simulink model "Drone_fuck_around"  (R2022a)
settings: Solver=VariableStepAuto  StartTime=0.0  StopTime=1  RelTol=1e-7  AbsTol=1e-8
model workspace: external: MATLAB File C:\Users\ivanb\OneDrive\Documents\Team 2261 Files\Mechanical Simulation\DroneMk1_DataFile1.m (data not in the file)
values from neighbouring files (symbols this model uses):
  smiData = saveVarsMat.smiData    [DroneMk1_DataFile1.m]    (also in DroneMk1_DataFile1.mat = )
undefined symbols (not defined in the file or in its folder): X, Y, Z
libraries: sm_lib x42, nesl_utility x30
(part 1 of 2)
settings Model: Creator=ivanb  LastModifiedBy=ivanb
settings SolverCC: InitialStep=1e-8  ZeroCrossAlgorithm=Adaptive

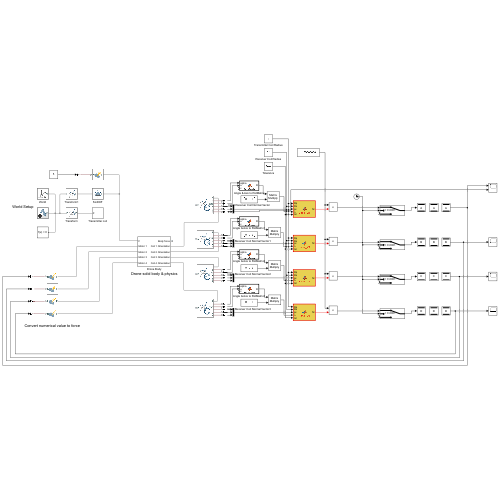
[thumbnail: Simulink's stored preview of the top-level diagram]
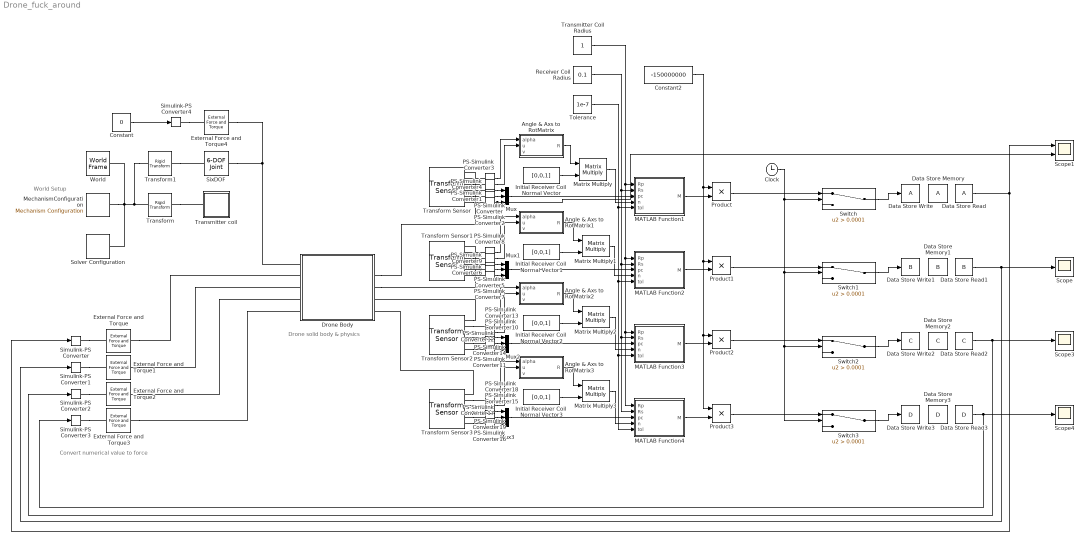
== system Drone_fuck_around ==
  note: Drone solid body & physics
  note: World Setup
  note: Convert numerical value to force
  Angle & Axs to RotMatrix : MATLAB Function  TreatAsAtomicUnit=on
  Angle & Axs to RotMatrix1 : MATLAB Function  TreatAsAtomicUnit=on
  Angle & Axs to RotMatrix2 : MATLAB Function  TreatAsAtomicUnit=on
  Angle & Axs to RotMatrix3 : MATLAB Function  TreatAsAtomicUnit=on
  Clock : Clock
  Constant : Constant  Value=0
  Constant2 : Constant  Value=-150000000
  Data Store Memory : DataStoreMemory  WriteAfterWriteMsg=warning  ShowAdditionalParam=off
  Data Store Memory1 : DataStoreMemory  DataStoreName=B  WriteAfterWriteMsg=warning  ShowAdditionalParam=off
  Data Store Memory2 : DataStoreMemory  DataStoreName=C  WriteAfterWriteMsg=warning  ShowAdditionalParam=off
  Data Store Memory3 : DataStoreMemory  DataStoreName=D  WriteAfterWriteMsg=warning  ShowAdditionalParam=off
  Data Store Read : DataStoreRead  IndexOptions=Index vector (dialog)  Indices=1  OutputSizes=1
  Data Store Read1 : DataStoreRead  DataStoreName=B  IndexOptions=Index vector (dialog)  Indices=1  OutputSizes=1
  Data Store Read2 : DataStoreRead  DataStoreName=C  IndexOptions=Index vector (dialog)  Indices=1  OutputSizes=1
  Data Store Read3 : DataStoreRead  DataStoreName=D  IndexOptions=Index vector (dialog)  Indices=1  OutputSizes=1
  Data Store Write : DataStoreWrite  IndexOptions=Index vector (dialog)  Indices=1  OutputSizes=1
  Data Store Write1 : DataStoreWrite  DataStoreName=B  IndexOptions=Index vector (dialog)  Indices=1  OutputSizes=1
  Data Store Write2 : DataStoreWrite  DataStoreName=C  IndexOptions=Index vector (dialog)  Indices=1  OutputSizes=1
  Data Store Write3 : DataStoreWrite  DataStoreName=D  IndexOptions=Index vector (dialog)  Indices=1  OutputSizes=1
  Drone Body : Subsystem
  External Force and Torque{,1..3} (4 alike) : sm_lib/Forces and Torques/External Force and Torque  ForceResolutionFrame=AttachedFrame  EnableForceX=off  EnableForceY=off  EnableForceZ=on  EnableForce=off  TorqueResolutionFrame=AttachedFrame  EnableTorqueX=off  EnableTorqueY=off  EnableTorqueZ=off  EnableTorque=off
  External Force and Torque4 : sm_lib/Forces and Torques/External Force and Torque  ForceResolutionFrame=AttachedFrame  EnableForceX=off  EnableForceY=off  EnableForceZ=off  EnableForce=off  TorqueResolutionFrame=AttachedFrame  EnableTorqueX=off  EnableTorqueY=on  EnableTorqueZ=off  EnableTorque=off
  Initial Receiver Coil Normal Vector{,1..3} (4 alike) : Constant  Value=[0,0,1]
  MATLAB Function1 : MATLAB Function  TreatAsAtomicUnit=on
  MATLAB Function2 : MATLAB Function  TreatAsAtomicUnit=on
  MATLAB Function3 : MATLAB Function  TreatAsAtomicUnit=on
  MATLAB Function4 : MATLAB Function  TreatAsAtomicUnit=on
  Matrix Multiply{,1..3} (4 alike) : Product  Multiplication=Matrix(*)
  MechanismConfiguration : sm_lib/Utilities/Mechanism Configuration  UniformGravity=Constant  GravityVector=[0 0 -9.80665]  GravityUnits=m/s^2  LinearizationDelta=0.001  JointModeTransitionNonlinearIterations=2
  Mux{,1..3} (4 alike) : Mux  Inputs=3
  PS-Simulink Converter{,1..19} (20 alike) : nesl_utility/PS-Simulink Converter  PhysicalDomain=network_engine_domain  SubClassName=ps_output  LeftPortType=input  RightPortType=output  PseudoPeriodic=off  Frequencies=[]  VectorFormat=inherit  Unit=inherit  AffineConversion=off
      settings: SourceProductBaseCode=SS,PW,VE
  Product{,1..3} (4 alike) : Product
  Receiver Coil Radius : Constant  Value=0.1
  Scope : Scope
  Scope1 : Scope  NumInputPorts=2
  Scope3 : Scope
  Scope4 : Scope
  Simulink-PS Converter{,1..4} (5 alike) : nesl_utility/Simulink-PS Converter  PhysicalDomain=network_engine_domain  SubClassName=ps_input  LeftPortType=input  RightPortType=output  PseudoPeriodic=off  Frequencies=[]  NoiseDistribution=none  NoiseParameters=[]  Unit=1  AffineConversion=off  FilteringAndDerivatives=provide  SimscapeFilterOrder=1  InputFilterTimeConstant=0.001  UdotUserProvided=0
      settings: SourceProductBaseCode=SS,PW,VE
  SixDOF : sm_lib/Joints/6-DOF Joint  JointMode=Normal  SenseConstraintForce=off  SenseConstraintForceX=off  SenseConstraintForceY=off  SenseConstraintForceZ=off  SenseConstraintTorque=off  SenseConstraintTorqueX=off  SenseConstraintTorqueY=off  SenseConstraintTorqueZ=off  SenseTotalForce=off  SenseTotalForceX=off  SenseTotalForceY=off  SenseTotalForceZ=off  SenseTotalTorque=off  SenseTotalTorqueX=off  SenseTotalTorqueY=off  SenseTotalTorqueZ=off  CompositeWrenchDir=FollowerOnBase  CompositeWrenchFrame=BaseFrame  PxEquilibriumPosition=0  PxEquilibriumPositionUnits=m  PxSpringStiffness=0  PxSpringStiffnessUnits=N/m  PxDampingCoefficient=0  PxDampingCoefficientUnits=N/(m/s)  PxTorqueActuationMode=NoTorque  PxMotionActuationMode=ComputedMotion  PxSensePosition=off  PxSenseVelocity=off  PxSenseAcceleration=off  PxSenseTorqueForce=off  PxSenseLowerLimitTorqueForce=off  PxSenseUpperLimitTorqueForce=off  PxLowerLimitSpecify=off  PxLowerLimitBound=-1  PxLowerLimitBoundUnits=m  PxLowerLimitStiffness=1e6  PxLowerLimitStiffnessUnits=N/m  PxLowerLimitDamping=1e3  PxLowerLimitDampingUnits=N/(m/s)  PxLowerLimitTransitionRegionWidth=1e-4  PxLowerLimitTransitionRegionWidthUnits=m  PxUpperLimitSpecify=off  PxUpperLimitBound=1  PxUpperLimitBoundUnits=m  PxUpperLimitStiffness=1e6  PxUpperLimitStiffnessUnits=N/m  PxUpperLimitDamping=1e3  PxUpperLimitDampingUnits=N/(m/s)  PxUpperLimitTransitionRegionWidth=1e-4  PxUpperLimitTransitionRegionWidthUnits=m  PxPositionTargetSpecify=off  PxPositionTargetPriority=High  PxPositionTargetValue=0  PxPositionTargetValueUnits=m  PxVelocityTargetSpecify=off  PxVelocityTargetPriority=High  PxVelocityTargetValue=0.001  PxVelocityTargetValueUnits=m/s  PyEquilibriumPosition=0  PyEquilibriumPositionUnits=m  PySpringStiffness=0  PySpringStiffnessUnits=N/m  PyDampingCoefficient=0  PyDampingCoefficientUnits=N/(m/s)  PyTorqueActuationMode=NoTorque  PyMotionActuationMode=ComputedMotion  PySensePosition=off  PySenseVelocity=off  PySenseAcceleration=off  PySenseTorqueForce=off  PySenseLowerLimitTorqueForce=off  PySenseUpperLimitTorqueForce=off  PyLowerLimitSpecify=off  PyLowerLimitBound=-1  PyLowerLimitBoundUnits=m  PyLowerLimitStiffness=1e6  PyLowerLimitStiffnessUnits=N/m  PyLowerLimitDamping=1e3  PyLowerLimitDampingUnits=N/(m/s)  PyLowerLimitTransitionRegionWidth=1e-4  PyLowerLimitTransitionRegionWidthUnits=m  PyUpperLimitSpecify=off  PyUpperLimitBound=1  PyUpperLimitBoundUnits=m  PyUpperLimitStiffness=1e6  PyUpperLimitStiffnessUnits=N/m  PyUpperLimitDamping=1e3  PyUpperLimitDampingUnits=N/(m/s)  PyUpperLimitTransitionRegionWidth=1e-4  PyUpperLimitTransitionRegionWidthUnits=m  PyPositionTargetSpecify=off  PyPositionTargetPriority=High  PyPositionTargetValue=0  PyPositionTargetValueUnits=m  PyVelocityTargetSpecify=off  PyVelocityTargetPriority=High  PyVelocityTargetValue=0  PyVelocityTargetValueUnits=m/s  PzEquilibriumPosition=0  PzEquilibriumPositionUnits=m  PzSpringStiffness=0  PzSpringStiffnessUnits=N/m  PzDampingCoefficient=0  PzDampingCoefficientUnits=N/(m/s)  PzTorqueActuationMode=NoTorque  PzMotionActuationMode=ComputedMotion  PzSensePosition=off  PzSenseVelocity=off  PzSenseAcceleration=off  PzSenseTorqueForce=off  PzSenseLowerLimitTorqueForce=off  PzSenseUpperLimitTorqueForce=off  PzLowerLimitSpecify=off  PzLowerLimitBound=-1  PzLowerLimitBoundUnits=m  PzLowerLimitStiffness=1e6  PzLowerLimitStiffnessUnits=N/m  PzLowerLimitDamping=1e3  PzLowerLimitDampingUnits=N/(m/s)  PzLowerLimitTransitionRegionWidth=1e-4  PzLowerLimitTransitionRegionWidthUnits=m  PzUpperLimitSpecify=off  PzUpperLimitBound=1  PzUpperLimitBoundUnits=m  PzUpperLimitStiffness=1e6  PzUpperLimitStiffnessUnits=N/m  PzUpperLimitDamping=1e3  PzUpperLimitDampingUnits=N/(m/s)  PzUpperLimitTransitionRegionWidth=1e-4  PzUpperLimitTransitionRegionWidthUnits=m  PzPositionTargetSpecify=off  PzPositionTargetPriority=High  PzPositionTargetValue=0  PzPositionTargetValueUnits=m  PzVelocityTargetSpecify=off  PzVelocityTargetPriority=High  PzVelocityTargetValue=0  PzVelocityTargetValueUnits=m/s  SphDefPosRotationMethod=None  SphDefPosRotationAngleUnits=deg  SphDefPosRotationStandardAxis=+Z  SphDefPosRotationAngle=0.0  SphDefPosRotationArbitraryAxis=[0 0 1]  SphDefPosFollAlignAxisA=+X  SphDefPosBaseAlignAxisA=+Y  SphDefPosFollAlignAxisB=+Y  SphDefPosBaseAlignAxisB=+Z  SphDefPosRotationSequenceAxes=FollowerAxes  SphDefPosRotationSequence=XYX  SphDefPosRotationSequenceAngles=[0 0 0]  SphDefPosRotationSequenceAnglesUnits=deg  SphDefPosRotationMatrix=[1 0 0; 0 1 0; 0 0 1]  SphEqPosRotationMethod=None  SphEqPosRotationAngleUnits=deg  SphEqPosRotationStandardAxis=+Z  SphEqPosRotationAngle=0.0  SphEqPosRotationArbitraryAxis=[0 0 1]  SphEqPosFollAlignAxisA=+X  SphEqPosBaseAlignAxisA=+Y  SphEqPosFollAlignAxisB=+Y  SphEqPosBaseAlignAxisB=+Z  SphEqPosRotationSequenceAxes=FollowerAxes  SphEqPosRotationSequence=XYX  SphEqPosRotationSequenceAngles=[0 0 0]  SphEqPosRotationSequenceAnglesUnits=deg  SphEqPosRotationMatrix=[1 0 0; 0 1 0; 0 0 1]  SphSpringStiffness=0  SphSpringStiffnessUnits=N*m/deg  SphDampingCoefficient=0  SphDampingCoefficientUnits=N*m/(deg/s)  SphActuateTorqueX=off  SphActuateTorqueY=off  SphActuateTorqueZ=off  SphActuateTorque=off  SphTorqueActuationMode=NoTorque  SphMotionActuationMode=ComputedMotion  SphActuationFrame=BaseFrame  SphSensePosition=off  SphSenseVelocityX=off  SphSenseVelocityY=off  SphSenseVelocityZ=off  SphSenseVelocity=off  SphSenseAccelerationX=off  SphSenseAccelerationY=off  SphSenseAccelerationZ=off  SphSenseAcceleration=off  SphSenseTorqueX=off  SphSenseTorqueY=off  SphSenseTorqueZ=off  SphSenseTorqueForce=off  SphSenseLowerLimitTorqueMag=off  SphSenseUpperLimitTorqueMag=off  SphSensingFrame=FollowerFrame  SphLowerLimitSpecify=off  SphLowerLimitBound=15  SphLowerLimitBoundUnits=deg  SphLowerLimitStiffness=1e4  SphLowerLimitStiffnessUnits=N*m/deg  SphLowerLimitDamping=10  SphLowerLimitDampingUnits=N*m/(deg/s)  SphLowerLimitTransitionRegionWidth=0.1  SphLowerLimitTransitionRegionWidthUnits=deg  SphUpperLimitSpecify=off  SphUpperLimitBound=45  SphUpperLimitBoundUnits=deg  SphUpperLimitStiffness=1e4  SphUpperLimitStiffnessUnits=N*m/deg  SphUpperLimitDamping=10  SphUpperLimitDampingUnits=N*m/(deg/s)  SphUpperLimitTransitionRegionWidth=0.1  SphUpperLimitTransitionRegionWidthUnits=deg  SphPositionTargetRotationMethod=None  SphPositionTargetRotationAngleUnits=deg  SphPositionTargetRotationStandardAxis=+Z  SphPositionTargetRotationAngle=0.0  SphPositionTargetRotationArbitraryAxis=[0 0 1]  SphPositionTargetFollAlignAxisA=+X  SphPositionTargetBaseAlignAxisA=+Y  SphPositionTargetFollAlignAxisB=+Y  SphPositionTargetBaseAlignAxisB=+Z  SphPositionTargetRotationSequenceAxes=FollowerAxes  SphPositionTargetRotationSequence=XYX  SphPositionTargetRotationSequenceAngles=[0 0 0]  SphPositionTargetRotationSequenceAnglesUnits=deg  SphPositionTargetRotationMatrix=[1 0 0; 0 1 0; 0 0 1]  SphPositionTargetSpecify=off  SphPositionTargetPriority=High  SphVelocityTargetValue=[0 0 0]  SphVelocityTargetValueUnits=deg/s  SphVelocityTargetSpecify=off  SphVelocityTargetPriority=High  SphVelocityTargetInFollowerFrame=on
  Solver Configuration : nesl_utility/Solver Configuration  PhysicalDomain=network_engine_domain  SubClassName=solver  LeftPortType=input  RightPortType=generic  Tones=[]  Harmonics=[]  SimulateNoise=off  Profile=off  UseLocalSampling=off  EnableSwitchedLinearOptims=on  FrequencyDomain=off  UseCCode=off  RelTol=0.001  AbsTol=0.001  MinStep=1e-09  ToWorkspace=off  RevertToSquareIcSolve=off  NumHomotopyIterations=100  PhasorMode=off  PhasorModeNumHarmonics=1  IndexReductionMethod=DerivativeReplacement  DoDC=off  ResidualTolerance=1e-09  UseLocalSolver=off  LocalSolverChoice=NE_BACKWARD_EULER_ADVANCER  LocalSolverSampleTime=0.001  DoFixedCost=off  MaxNonlinIter=3  MaxModeIter=2  ComputeImpulses=off  ImpulseIterations=2  LinearAlgebra=auto  LinearAlgebraNumThread=0  EquationFormulation=NE_TIME_EF  DelaysMemoryBudget=1024  AutomaticFiltering=on  FilteringTimeConstant=0.001  PartitionStorageMethod=AS_NEEDED  PartitionMemoryBudget=1024  PartitionMethod=ROBUST
      settings: SourceProductBaseCode=SS,PW,VE
  Switch{,1..3} (4 alike) : Switch  Criteria=u2 > Threshold  Threshold=0.0001  SaturateOnIntegerOverflow=off  InputSameDT=off
  Tolerance : Constant  Value=1e-7
  Transform : sm_lib/Frames and Transforms/Rigid Transform  TranslationMethod=Cartesian  TranslationStandardOffset=0  TranslationLengthUnit=m  TranslationStandardAxis=+Z  TranslationCartesianOffset=[0, 0, 0]  TranslationROffset=0  TranslationROffsetUnits=m  TranslationZOffset=0  TranslationZOffsetUnits=m  TranslationThetaOffset=0  TranslationThetaOffsetUnits=deg  RotationMethod=StandardAxis  RotationAngleUnits=rad  RotationStandardAxis=-X  RotationAngle=pi/2  RotationArbitraryAxis=smiData.RigidTransform(1).axis  FollAlignAxisA=+X  BaseAlignAxisA=+Y  FollAlignAxisB=+Y  BaseAlignAxisB=+Z  RotationSequenceAxes=FollowerAxes  RotationSequence=XYX  RotationSequenceAngles=[0 0 0]  RotationSequenceAnglesUnits=deg  RotationMatrix=[1 0 0; 0 1 0; 0 0 1]
  Transform Sensor{,1..3} (4 alike) : sm_lib/Frames and Transforms/Transform Sensor  MeasurementFrame=World  SenseAngle=on  SenseAxis=on  SenseAngle1=off  SenseAngle2=off  SenseAngle3=off  SenseQ=off  SenseR=off  SenseOmegaX=off  SenseOmegaY=off  SenseOmegaZ=off  SenseOmega1=off  SenseOmega2=off  SenseOmega3=off  SenseQDot=off  SenseRDot=off  SenseAlphaX=off  SenseAlphaY=off  SenseAlphaZ=off  SenseAlpha1=off  SenseAlpha2=off  SenseAlpha3=off  SenseQDDot=off  SenseRDDot=off  SenseX=on  SenseY=on  SenseZ=on  SenseRad=off  SenseAzim=off  SenseDist=off  SenseInc=off  SenseXDot=off  SenseYDot=off  SenseZDot=off  SenseRadDot=off  SenseAzimDot=off  SenseDistDot=off  SenseIncDot=off  SenseXDDot=off  SenseYDDot=off  SenseZDDot=off  SenseRadDDot=off  SenseAzimDDot=off  SenseDistDDot=off  SenseIncDDot=off
  Transform1 : sm_lib/Frames and Transforms/Rigid Transform  TranslationMethod=Cartesian  TranslationStandardOffset=0  TranslationLengthUnit=m  TranslationStandardAxis=+Z  TranslationCartesianOffset=[0, 0, 0.1]  TranslationROffset=0  TranslationROffsetUnits=m  TranslationZOffset=0  TranslationZOffsetUnits=m  TranslationThetaOffset=0  TranslationThetaOffsetUnits=deg  RotationMethod=StandardAxis  RotationAngleUnits=rad  RotationStandardAxis=+X  RotationAngle=pi/2  RotationArbitraryAxis=smiData.RigidTransform(2).axis  FollAlignAxisA=+X  BaseAlignAxisA=+Y  FollAlignAxisB=+Y  BaseAlignAxisB=+Z  RotationSequenceAxes=FollowerAxes  RotationSequence=XYX  RotationSequenceAngles=[0 0 0]  RotationSequenceAnglesUnits=deg  RotationMatrix=[1 0 0; 0 1 0; 0 0 1]
  Transmitter Coil Radius : Constant
  Transmitter coil : Subsystem
  World : sm_lib/Frames and Transforms/World Frame
  wires:
  Switch/1 -> Data Store Write/1
  Clock/1 -> Switch3/2, Switch2/2, Switch1/2, Switch/2
  Data Store Read/1 -> Simulink-PS Converter/1, Scope1/1
  Mux3/1 -> MATLAB Function4/3(pc)
  Matrix Multiply1/1 -> MATLAB Function2/4(n)
  Angle & Axs to RotMatrix1/1(R) -> Matrix Multiply1/1
  MATLAB Function2/1(M) -> Product1/2
  PS-Simulink Converter12/1 -> Mux2/3
  PS-Simulink Converter10/1 -> Mux2/1
  Initial Receiver Coil Normal Vector3/1 -> Matrix Multiply3/2
  PS-Simulink Converter3/1 -> Angle & Axs to RotMatrix/1(alpha)
  MATLAB Function3/1(M) -> Product2/2
  PS-Simulink Converter18/1 -> Angle & Axs to RotMatrix3/1(alpha)
  Initial Receiver Coil Normal Vector2/1 -> Matrix Multiply2/2
  Receiver Coil Radius/1 -> MATLAB Function1/2(Rs), MATLAB Function2/2(Rs), MATLAB Function4/2(Rs), MATLAB Function3/2(Rs)
  Tolerance/1 -> MATLAB Function1/5(tol), MATLAB Function2/5(tol), MATLAB Function4/5(tol), MATLAB Function3/5(tol)
  Initial Receiver Coil Normal Vector1/1 -> Matrix Multiply1/2
  MATLAB Function4/1(M) -> Product3/2
  PS-Simulink Converter19/1 -> Angle & Axs to RotMatrix3/2(u)
  Transmitter Coil Radius/1 -> MATLAB Function1/1(Rp), MATLAB Function2/1(Rp), MATLAB Function4/1(Rp), MATLAB Function3/1(Rp)
  Angle & Axs to RotMatrix3/1(R) -> Matrix Multiply3/1
  PS-Simulink Converter6/1 -> Mux1/2
  Initial Receiver Coil Normal Vector/1 -> Matrix Multiply/2
  Matrix Multiply3/1 -> MATLAB Function4/4(n)
  PS-Simulink Converter14/1 -> Angle & Axs to RotMatrix2/2(u)
  PS-Simulink Converter9/1 -> Angle & Axs to RotMatrix1/2(u)
  PS-Simulink Converter7/1 -> Mux1/3
  PS-Simulink Converter13/1 -> Angle & Axs to RotMatrix2/1(alpha)
  PS-Simulink Converter17/1 -> Mux3/3
  PS-Simulink Converter2/1 -> Scope1/2, Mux/3
  PS-Simulink Converter16/1 -> Mux3/2
  PS-Simulink Converter15/1 -> Mux3/1
  Mux2/1 -> MATLAB Function3/3(pc)
  MATLAB Function1/1(M) -> Product/2
  PS-Simulink Converter8/1 -> Angle & Axs to RotMatrix1/1(alpha)
  Mux1/1 -> MATLAB Function2/3(pc)
  Angle & Axs to RotMatrix/1(R) -> Matrix Multiply/1
  PS-Simulink Converter11/1 -> Mux2/2
  Constant/1 -> Simulink-PS Converter4/1
  Mux/1 -> MATLAB Function1/3(pc)
  PS-Simulink Converter4/1 -> Angle & Axs to RotMatrix/2(u)
  Angle & Axs to RotMatrix2/1(R) -> Matrix Multiply2/1
  Matrix Multiply/1 -> MATLAB Function1/4(n)
  PS-Simulink Converter/1 -> Mux/1
  Matrix Multiply2/1 -> MATLAB Function3/4(n)
  PS-Simulink Converter5/1 -> Mux1/1
  Switch1/1 -> Data Store Write1/1
  Switch2/1 -> Data Store Write2/1
  Switch3/1 -> Data Store Write3/1
  Data Store Read1/1 -> Scope/1, Simulink-PS Converter1/1
  Data Store Read2/1 -> Scope3/1, Simulink-PS Converter2/1
  Data Store Read3/1 -> Scope4/1, Simulink-PS Converter3/1
  Constant2/1 -> Product3/1, Product2/1, Product1/1, Product/1
  PS-Simulink Converter1/1 -> Mux/2
  Product/1 -> Switch/1
  Product1/1 -> Switch1/1
  Product2/1 -> Switch2/1
  Product3/1 -> Switch3/1
  connections:
  Transform1/LConn1 -- Transform/LConn1 -- MechanismConfiguration/RConn1 -- Solver Configuration/RConn1 -- World/RConn1
  SixDOF/RConn1 -- Drone Body/LConn1 -- External Force and Torque4/RConn1
  Transform Sensor2/RConn2 -- PS-Simulink Converter13/LConn1
  Transform Sensor3/RConn5 -- PS-Simulink Converter16/LConn1
  Transform Sensor3/RConn3 -- PS-Simulink Converter19/LConn1
  External Force and Torque2/RConn1 -- Drone Body/LConn4
  Transform Sensor3/RConn6 -- PS-Simulink Converter17/LConn1
  Transform Sensor2/RConn1 -- Drone Body/RConn4
  Transform Sensor/RConn3 -- PS-Simulink Converter4/LConn1
  Simulink-PS Converter4/RConn1 -- External Force and Torque4/LConn1
  Drone Body/RConn2 -- Transform Sensor/RConn1
  Simulink-PS Converter3/RConn1 -- External Force and Torque3/LConn1
  Transform Sensor1/RConn2 -- PS-Simulink Converter8/LConn1
  Transform Sensor/RConn2 -- PS-Simulink Converter3/LConn1
  Transform Sensor1/RConn5 -- PS-Simulink Converter6/LConn1
  Transform Sensor2/RConn3 -- PS-Simulink Converter14/LConn1
  Simulink-PS Converter/RConn1 -- External Force and Torque/LConn1
  Transform Sensor/RConn5 -- PS-Simulink Converter1/LConn1
  External Force and Torque3/RConn1 -- Drone Body/LConn5
  Transform Sensor1/RConn3 -- PS-Simulink Converter9/LConn1
  Drone Body/RConn3 -- Transform Sensor1/RConn1
  Transform Sensor3/RConn4 -- PS-Simulink Converter15/LConn1
  Transform Sensor3/RConn2 -- PS-Simulink Converter18/LConn1
  Transform Sensor/RConn6 -- PS-Simulink Converter2/LConn1
  Simulink-PS Converter1/RConn1 -- External Force and Torque1/LConn1
  Transform Sensor1/RConn6 -- PS-Simulink Converter7/LConn1
  Transform Sensor3/RConn1 -- Drone Body/RConn5
  External Force and Torque/RConn1 -- Drone Body/LConn2
  Transform Sensor2/RConn4 -- PS-Simulink Converter10/LConn1
  Transform Sensor/RConn4 -- PS-Simulink Converter/LConn1
  Transform/RConn1 -- Transmitter coil/LConn1
  Transform Sensor2/RConn5 -- PS-Simulink Converter11/LConn1
  Simulink-PS Converter2/RConn1 -- External Force and Torque2/LConn1
  Transform Sensor2/RConn6 -- PS-Simulink Converter12/LConn1
  Transform Sensor1/RConn4 -- PS-Simulink Converter5/LConn1
  External Force and Torque1/RConn1 -- Drone Body/LConn3
  Transform1/RConn1 -- SixDOF/LConn1

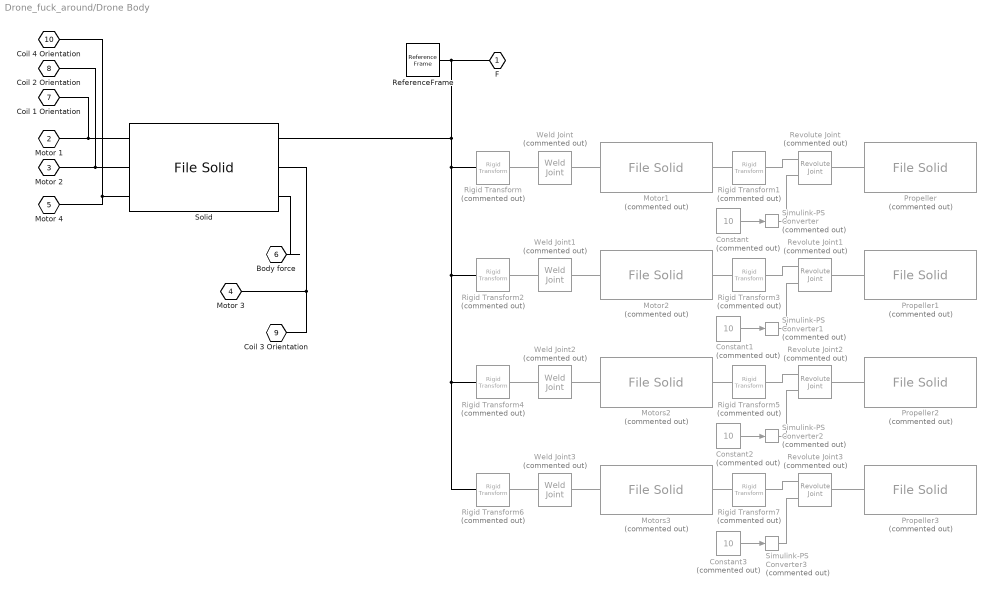
== system Drone_fuck_around/Drone Body ==
  Constant{,1..3} (4 alike) : Constant  Commented=on  Value=10
  Motor1 : sm_lib/Body Elements/File Solid  Commented=on  ExtGeomFileName=C:\Users\ivanb\OneDrive\Documents\Team 2261 Files\Mechanical Simulation\Drone Rendering\Rendered_for_simulink\DC_MOTOR_(Brushless DC Inrunner Motor)_Default_sldprt.STEP  UnitType=FromFile  ExtGeomFileUnits=m  StepReaderType=HEX  ExportConvexHullGeometry=off  InertiaType=CalculateFromGeometry  Mass=1  MassUnits=kg  CenterOfMass=[0 0 0]  CenterOfMassUnits=m  MomentsOfInertia=[1 1 1]  MomentsOfInertiaUnits=kg*m^2  ProductsOfInertia=[0 0 0]  ProductsOfInertiaUnits=kg*m^2  BasedOnType=Density  Density=1000  DensityUnits=kg/m^3  DoExposeReferenceFrame=on  SerializedFrames=<Frames><Frame><Id>Frame1</Id><Value><Name>Position</Name><Origin><Source>ReferenceFrame</Source><FeatureName></FeatureName></Origin><PrimaryAxis><DefinedDirection>+Z</DefinedDirection><Source>ReferenceFrame</Source><SourceDirection>+Z</SourceDirection><FeatureName></FeatureName></PrimaryAxis><SecondaryAxis><DefinedDirection>+X</DefinedDirection><Source>ReferenceFrame</Source><SourceDirection>+X</SourceDirection><FeatureName></FeatureName></SecondaryAxis></Value></Frame></Frames>  GraphicType=FromGeometry  MarkerShape=Sphere  MarkerSize=10  GraphicVisPropType=SimpleVisualProperties  GraphicDiffuseColor=[0.5 0.5 0.5]  GraphicSpecularColor=[0.5 0.5 0.5 1.0]  GraphicAmbientColor=[0.15 0.15 0.15 1.0]  GraphicEmissiveColor=[0.0 0.0 0.0 1.0]  GraphicShininess=75  GraphicOpacity=1.0
  Motor2 : sm_lib/Body Elements/File Solid  Commented=on  ExtGeomFileName=C:\Users\ivanb\OneDrive\Documents\Team 2261 Files\Mechanical Simulation\Drone Rendering\Rendered_for_simulink\DC_MOTOR_(Brushless DC Inrunner Motor)_Default_sldprt.STEP  UnitType=FromFile  ExtGeomFileUnits=m  StepReaderType=HEX  ExportConvexHullGeometry=off  InertiaType=CalculateFromGeometry  Mass=1  MassUnits=kg  CenterOfMass=[0 0 0]  CenterOfMassUnits=m  MomentsOfInertia=[1 1 1]  MomentsOfInertiaUnits=kg*m^2  ProductsOfInertia=[0 0 0]  ProductsOfInertiaUnits=kg*m^2  BasedOnType=Density  Density=1000  DensityUnits=kg/m^3  DoExposeReferenceFrame=on  SerializedFrames=<Frames><Frame><Id>Frame1</Id><Value><Name>Position</Name><Origin><Source>ReferenceFrame</Source><FeatureName></FeatureName></Origin><PrimaryAxis><DefinedDirection>+Z</DefinedDirection><Source>ReferenceFrame</Source><SourceDirection>+Z</SourceDirection><FeatureName></FeatureName></PrimaryAxis><SecondaryAxis><DefinedDirection>+X</DefinedDirection><Source>ReferenceFrame</Source><SourceDirection>+X</SourceDirection><FeatureName></FeatureName></SecondaryAxis></Value></Frame></Frames>  GraphicType=FromGeometry  MarkerShape=Sphere  MarkerSize=10  GraphicVisPropType=SimpleVisualProperties  GraphicDiffuseColor=[0.5 0.5 0.5]  GraphicSpecularColor=[0.5 0.5 0.5 1.0]  GraphicAmbientColor=[0.15 0.15 0.15 1.0]  GraphicEmissiveColor=[0.0 0.0 0.0 1.0]  GraphicShininess=75  GraphicOpacity=1.0
  Motors2 : sm_lib/Body Elements/File Solid  Commented=on  ExtGeomFileName=C:\Users\ivanb\OneDrive\Documents\Team 2261 Files\Mechanical Simulation\Drone Rendering\Rendered_for_simulink\DC_MOTOR_(Brushless DC Inrunner Motor)_Default_sldprt.STEP  UnitType=FromFile  ExtGeomFileUnits=m  StepReaderType=HEX  ExportConvexHullGeometry=off  InertiaType=CalculateFromGeometry  Mass=1  MassUnits=kg  CenterOfMass=[0 0 0]  CenterOfMassUnits=m  MomentsOfInertia=[1 1 1]  MomentsOfInertiaUnits=kg*m^2  ProductsOfInertia=[0 0 0]  ProductsOfInertiaUnits=kg*m^2  BasedOnType=Density  Density=1000  DensityUnits=kg/m^3  DoExposeReferenceFrame=on  SerializedFrames=<Frames><Frame><Id>Frame1</Id><Value><Name>Position</Name><Origin><Source>ReferenceFrame</Source><FeatureName></FeatureName></Origin><PrimaryAxis><DefinedDirection>+Z</DefinedDirection><Source>ReferenceFrame</Source><SourceDirection>+Z</SourceDirection><FeatureName></FeatureName></PrimaryAxis><SecondaryAxis><DefinedDirection>+X</DefinedDirection><Source>ReferenceFrame</Source><SourceDirection>+X</SourceDirection><FeatureName></FeatureName></SecondaryAxis></Value></Frame></Frames>  GraphicType=FromGeometry  MarkerShape=Sphere  MarkerSize=10  GraphicVisPropType=SimpleVisualProperties  GraphicDiffuseColor=[0.5 0.5 0.5]  GraphicSpecularColor=[0.5 0.5 0.5 1.0]  GraphicAmbientColor=[0.15 0.15 0.15 1.0]  GraphicEmissiveColor=[0.0 0.0 0.0 1.0]  GraphicShininess=75  GraphicOpacity=1.0
  Motors3 : sm_lib/Body Elements/File Solid  Commented=on  ExtGeomFileName=C:\Users\ivanb\OneDrive\Documents\Team 2261 Files\Mechanical Simulation\Drone Rendering\Rendered_for_simulink\DC_MOTOR_(Brushless DC Inrunner Motor)_Default_sldprt.STEP  UnitType=FromFile  ExtGeomFileUnits=m  StepReaderType=HEX  ExportConvexHullGeometry=off  InertiaType=CalculateFromGeometry  Mass=1  MassUnits=kg  CenterOfMass=[0 0 0]  CenterOfMassUnits=m  MomentsOfInertia=[1 1 1]  MomentsOfInertiaUnits=kg*m^2  ProductsOfInertia=[0 0 0]  ProductsOfInertiaUnits=kg*m^2  BasedOnType=Density  Density=1000  DensityUnits=kg/m^3  DoExposeReferenceFrame=on  SerializedFrames=<Frames><Frame><Id>Frame1</Id><Value><Name>Position</Name><Origin><Source>ReferenceFrame</Source><FeatureName></FeatureName></Origin><PrimaryAxis><DefinedDirection>+Z</DefinedDirection><Source>ReferenceFrame</Source><SourceDirection>+Z</SourceDirection><FeatureName></FeatureName></PrimaryAxis><SecondaryAxis><DefinedDirection>+X</DefinedDirection><Source>ReferenceFrame</Source><SourceDirection>+X</SourceDirection><FeatureName></FeatureName></SecondaryAxis></Value></Frame></Frames>  GraphicType=FromGeometry  MarkerShape=Sphere  MarkerSize=10  GraphicVisPropType=SimpleVisualProperties  GraphicDiffuseColor=[0.5 0.5 0.5]  GraphicSpecularColor=[0.5 0.5 0.5 1.0]  GraphicAmbientColor=[0.15 0.15 0.15 1.0]  GraphicEmissiveColor=[0.0 0.0 0.0 1.0]  GraphicShininess=75  GraphicOpacity=1.0
  Propeller{,1..3} (4 alike) : sm_lib/Body Elements/File Solid  Commented=on  ExtGeomFileName=C:\Users\ivanb\OneDrive\Documents\Team 2261 Files\Mechanical Simulation\Drone Rendering\Rendered_for_simulink\Propeller_Default_sldprt.STEP  UnitType=FromFile  ExtGeomFileUnits=m  StepReaderType=HEX  ExportConvexHullGeometry=off  InertiaType=CalculateFromGeometry  Mass=1  MassUnits=kg  CenterOfMass=[0 0 0]  CenterOfMassUnits=m  MomentsOfInertia=[1 1 1]  MomentsOfInertiaUnits=kg*m^2  ProductsOfInertia=[0 0 0]  ProductsOfInertiaUnits=kg*m^2  BasedOnType=Density  Density=1000  DensityUnits=kg/m^3  DoExposeReferenceFrame=on  SerializedFrames=<Frames><Frame><Id>Frame1</Id><Value><Name>Rotation point</Name><Origin><Source>ReferenceFrame</Source><FeatureName></FeatureName></Origin><PrimaryAxis><DefinedDirection>+Z</DefinedDirection><Source>ReferenceFrame</Source><SourceDirection>+Z</SourceDirection><FeatureName></FeatureName></PrimaryAxis><SecondaryAxis><DefinedDirection>+X</DefinedDirection><Source>ReferenceFrame</Source><SourceDirection>+X</SourceDirection><FeatureName></FeatureName></SecondaryAxis></Value></Frame></Frames>  GraphicType=FromGeometry  MarkerShape=Sphere  MarkerSize=10  GraphicVisPropType=SimpleVisualProperties  GraphicDiffuseColor=[0.5 0.5 0.5]  GraphicSpecularColor=[0.5 0.5 0.5 1.0]  GraphicAmbientColor=[0.15 0.15 0.15 1.0]  GraphicEmissiveColor=[0.0 0.0 0.0 1.0]  GraphicShininess=75  GraphicOpacity=1.0
  ReferenceFrame : sm_lib/Frames and Transforms/Reference Frame
  Revolute Joint{,1..3} (4 alike) : sm_lib/Joints/Revolute Joint  Commented=on  JointMode=Normal  SenseConstraintForce=off  SenseConstraintForceX=off  SenseConstraintForceY=off  SenseConstraintForceZ=off  SenseConstraintTorque=off  SenseConstraintTorqueX=off  SenseConstraintTorqueY=off  SenseConstraintTorqueZ=off  SenseTotalForce=off  SenseTotalForceX=off  SenseTotalForceY=off  SenseTotalForceZ=off  SenseTotalTorque=off  SenseTotalTorqueX=off  SenseTotalTorqueY=off  SenseTotalTorqueZ=off  CompositeWrenchDir=FollowerOnBase  CompositeWrenchFrame=BaseFrame  EquilibriumPosition=0  EquilibriumPositionUnits=deg  SpringStiffness=0  SpringStiffnessUnits=N*m/deg  DampingCoefficient=0.001  DampingCoefficientUnits=N*m/(deg/s)  TorqueActuationMode=InputTorque  MotionActuationMode=ComputedMotion  SensePosition=off  SenseVelocity=off  SenseAcceleration=off  SenseTorqueForce=off  SenseLowerLimitTorqueForce=off  SenseUpperLimitTorqueForce=off  LowerLimitSpecify=off  LowerLimitBound=-90  LowerLimitBoundUnits=deg  LowerLimitStiffness=1e4  LowerLimitStiffnessUnits=N*m/deg  LowerLimitDamping=10  LowerLimitDampingUnits=N*m/(deg/s)  LowerLimitTransitionRegionWidth=0.1  LowerLimitTransitionRegionWidthUnits=deg  UpperLimitSpecify=off  UpperLimitBound=90  UpperLimitBoundUnits=deg  UpperLimitStiffness=1e4  UpperLimitStiffnessUnits=N*m/deg  UpperLimitDamping=10  UpperLimitDampingUnits=N*m/(deg/s)  UpperLimitTransitionRegionWidth=0.1  UpperLimitTransitionRegionWidthUnits=deg  PositionTargetSpecify=off  PositionTargetPriority=High  PositionTargetValue=0  PositionTargetValueUnits=deg  VelocityTargetSpecify=off  VelocityTargetPriority=Low  VelocityTargetValue=0  VelocityTargetValueUnits=rad/s
  Rigid Transform : sm_lib/Frames and Transforms/Rigid Transform  Commented=on  TranslationMethod=Cartesian  TranslationStandardOffset=0  TranslationLengthUnit=in  TranslationStandardAxis=+Z  TranslationCartesianOffset=[-2.42 2.32 -2.42]  TranslationROffset=0  TranslationROffsetUnits=m  TranslationZOffset=0  TranslationZOffsetUnits=m  TranslationThetaOffset=0  TranslationThetaOffsetUnits=deg  RotationMethod=StandardAxis  RotationAngleUnits=deg  RotationStandardAxis=+Z  RotationAngle=90  RotationArbitraryAxis=[0 0 1]  FollAlignAxisA=+X  BaseAlignAxisA=+Y  FollAlignAxisB=+Y  BaseAlignAxisB=+Z  RotationSequenceAxes=FollowerAxes  RotationSequence=XYX  RotationSequenceAngles=[0 0 0]  RotationSequenceAnglesUnits=deg  RotationMatrix=[1 0 0; 0 1 0; 0 0 1]
  Rigid Transform{1,3,5,7} (4 alike) : sm_lib/Frames and Transforms/Rigid Transform  Commented=on  TranslationMethod=Cartesian  TranslationStandardOffset=0  TranslationLengthUnit=in  TranslationStandardAxis=+Z  TranslationCartesianOffset=[-0.95 0 0]  TranslationROffset=0  TranslationROffsetUnits=m  TranslationZOffset=0  TranslationZOffsetUnits=m  TranslationThetaOffset=0  TranslationThetaOffsetUnits=deg  RotationMethod=StandardAxis  RotationAngleUnits=deg  RotationStandardAxis=+Y  RotationAngle=90  RotationArbitraryAxis=[0 0 1]  FollAlignAxisA=+X  BaseAlignAxisA=+Y  FollAlignAxisB=+Y  BaseAlignAxisB=+Z  RotationSequenceAxes=FollowerAxes  RotationSequence=XYX  RotationSequenceAngles=[0 0 0]  RotationSequenceAnglesUnits=deg  RotationMatrix=[1 0 0; 0 1 0; 0 0 1]
  Rigid Transform2 : sm_lib/Frames and Transforms/Rigid Transform  Commented=on  TranslationMethod=Cartesian  TranslationStandardOffset=0  TranslationLengthUnit=in  TranslationStandardAxis=+Z  TranslationCartesianOffset=[2.42 2.32 -2.42]  TranslationROffset=0  TranslationROffsetUnits=m  TranslationZOffset=0  TranslationZOffsetUnits=m  TranslationThetaOffset=0  TranslationThetaOffsetUnits=deg  RotationMethod=StandardAxis  RotationAngleUnits=deg  RotationStandardAxis=+Z  RotationAngle=90  RotationArbitraryAxis=[0 0 1]  FollAlignAxisA=+X  BaseAlignAxisA=+Y  FollAlignAxisB=+Y  BaseAlignAxisB=+Z  RotationSequenceAxes=FollowerAxes  RotationSequence=XYX  RotationSequenceAngles=[0 0 0]  RotationSequenceAnglesUnits=deg  RotationMatrix=[1 0 0; 0 1 0; 0 0 1]
  Rigid Transform4 : sm_lib/Frames and Transforms/Rigid Transform  Commented=on  TranslationMethod=Cartesian  TranslationStandardOffset=0  TranslationLengthUnit=in  TranslationStandardAxis=+Z  TranslationCartesianOffset=[-2.42 2.32 2.42]  TranslationROffset=0  TranslationROffsetUnits=m  TranslationZOffset=0  TranslationZOffsetUnits=m  TranslationThetaOffset=0  TranslationThetaOffsetUnits=deg  RotationMethod=StandardAxis  RotationAngleUnits=deg  RotationStandardAxis=+Z  RotationAngle=90  RotationArbitraryAxis=[0 0 1]  FollAlignAxisA=+X  BaseAlignAxisA=+Y  FollAlignAxisB=+Y  BaseAlignAxisB=+Z  RotationSequenceAxes=FollowerAxes  RotationSequence=XYX  RotationSequenceAngles=[0 0 0]  RotationSequenceAnglesUnits=deg  RotationMatrix=[1 0 0; 0 1 0; 0 0 1]
  Rigid Transform6 : sm_lib/Frames and Transforms/Rigid Transform  Commented=on  TranslationMethod=Cartesian  TranslationStandardOffset=0  TranslationLengthUnit=in  TranslationStandardAxis=+Z  TranslationCartesianOffset=[2.42 2.32 2.42]  TranslationROffset=0  TranslationROffsetUnits=m  TranslationZOffset=0  TranslationZOffsetUnits=m  TranslationThetaOffset=0  TranslationThetaOffsetUnits=deg  RotationMethod=StandardAxis  RotationAngleUnits=deg  RotationStandardAxis=+Z  RotationAngle=90  RotationArbitraryAxis=[0 0 1]  FollAlignAxisA=+X  BaseAlignAxisA=+Y  FollAlignAxisB=+Y  BaseAlignAxisB=+Z  RotationSequenceAxes=FollowerAxes  RotationSequence=XYX  RotationSequenceAngles=[0 0 0]  RotationSequenceAnglesUnits=deg  RotationMatrix=[1 0 0; 0 1 0; 0 0 1]
  Simulink-PS Converter{,1..3} (4 alike) : nesl_utility/Simulink-PS Converter  Commented=on  PhysicalDomain=network_engine_domain  SubClassName=ps_input  LeftPortType=input  RightPortType=output  PseudoPeriodic=off  Frequencies=[]  NoiseDistribution=none  NoiseParameters=[]  Unit=1  AffineConversion=off  FilteringAndDerivatives=provide  SimscapeFilterOrder=1  InputFilterTimeConstant=0.001  UdotUserProvided=0
      settings: SourceProductBaseCode=SS,PW,VE
  Solid : sm_lib/Body Elements/File Solid  ExtGeomFileName=C:\Users\ivanb\OneDrive\Documents\Team 2261 Files\Mechanical Simulation\Drone Rendering\Rendered_for_simulink\Drone render_Default_sldprt.STEP  UnitType=FromFile  ExtGeomFileUnits=m  StepReaderType=HEX  ExportConvexHullGeometry=off  InertiaType=CalculateFromGeometry  Mass=smiData.Solid(1).mass  MassUnits=kg  CenterOfMass=smiData.Solid(1).CoM  CenterOfMassUnits=in  MomentsOfInertia=smiData.Solid(1).MoI  MomentsOfInertiaUnits=kg*in^2  ProductsOfInertia=smiData.Solid(1).PoI  ProductsOfInertiaUnits=kg*in^2  BasedOnType=Density  Density=300  DensityUnits=kg/m^3  DoExposeReferenceFrame=on  SerializedFrames=<Frames><Frame><Id>Frame1</Id><Value><Name>Motor 1</Name><Origin><Source>GeometricFeature</Source><FeatureName>point 566</FeatureName></Origin><PrimaryAxis><DefinedDirection>+Z</DefinedDirection><Source>ReferenceFrame</Source><SourceDirection>+Z</SourceDirection><FeatureName></FeatureName></PrimaryAxis><SecondaryAxis><DefinedDirection>+X</DefinedDirection><Source>ReferenceFrame</Source><SourceDirection>+X</SourceDirection><FeatureName></FeatureName></SecondaryAxis></Value></Frame><Frame><Id>Frame2</Id><Value><Name>Motor 2</Name><Origin><Source>GeometricFeature</Source><FeatureName>point 537</FeatureName></Origin><PrimaryAxis><DefinedDirection>+Z</DefinedDirection><Source>ReferenceFrame</Source><SourceDirection>+Z</SourceDirection><FeatureName></FeatureName></PrimaryAxis><SecondaryAxis><DefinedDirection>+X</DefinedDirection><Source>ReferenceFrame</Source><SourceDirection>+X</SourceDirection><FeatureName></FeatureName></SecondaryAxis></Value></Frame><Frame><Id>Frame3</Id><Value><Name>Motor 3</Name><Origin><Source>GeometricFeature</Source><FeatureName>point 589</FeatureName></Origin><PrimaryAxis><DefinedDirection>+Z</DefinedDirection><Source>ReferenceFrame</Source><SourceDirection>+Z</SourceDirection><FeatureName></FeatureName></PrimaryAxis><SecondaryAxis><DefinedDirection>+X</DefinedDirection><Source>ReferenceFrame</Source><SourceDirection>+X</SourceDirection><FeatureName></FeatureName></SecondaryAxis></Value></Frame><Frame><Id>Frame4</Id><Value><Name>Motor 4</Name><Origin><Source>GeometricFeature</Source><FeatureName>point 618</FeatureName></Origin><PrimaryAxis><DefinedDirection>+Z</DefinedDirection><Source>ReferenceFrame</Source><SourceDirection>+Z</SourceDirection><FeatureName></FeatureName></PrimaryAxis><SecondaryAxis><DefinedDirection>+X</DefinedDirection><Source>ReferenceFrame</Source><SourceDirection>+X</SourceDirection><FeatureName></FeatureName></SecondaryAxis></Value></Frame><Frame><Id>Frame5</Id><Value><Name>Body</Name><Origin><Source>CenterOfMassFrame</Source><FeatureName></FeatureName></Origin><PrimaryAxis><DefinedDirection>+Z</DefinedDirection><Source>ReferenceFrame</Source><SourceDirection>+Z</SourceDirection><FeatureName></FeatureName></PrimaryAxis><SecondaryAxis><DefinedDirection>+X</DefinedDirection><Source>ReferenceFrame</Source><SourceDirection>+X</SourceDirection><FeatureName></FeatureName></SecondaryAxis></Value></Frame></Frames>  GraphicType=FromGeometry  MarkerShape=Sphere  MarkerSize=10  GraphicVisPropType=SimpleVisualProperties  GraphicDiffuseColor=smiData.Solid(1).color  GraphicSpecularColor=[0.5 0.5 0.5 1.0]  GraphicAmbientColor=[0.15 0.15 0.15 1.0]  GraphicEmissiveColor=[0.0 0.0 0.0 1.0]  GraphicShininess=75  GraphicOpacity=smiData.Solid(1).opacity
  Weld Joint{,1..3} (4 alike) : sm_lib/Joints/Weld Joint  Commented=on  JointMode=Normal  SenseConstraintForce=off  SenseConstraintForceX=off  SenseConstraintForceY=off  SenseConstraintForceZ=off  SenseConstraintTorque=off  SenseConstraintTorqueX=off  SenseConstraintTorqueY=off  SenseConstraintTorqueZ=off  SenseTotalForce=off  SenseTotalForceX=off  SenseTotalForceY=off  SenseTotalForceZ=off  SenseTotalTorque=off  SenseTotalTorqueX=off  SenseTotalTorqueY=off  SenseTotalTorqueZ=off  CompositeWrenchDir=FollowerOnBase  CompositeWrenchFrame=BaseFrame
  F : PMIOPort  Side=Left
  Motor 1 : PMIOPort  Port=2  Side=Left
  Motor 2 : PMIOPort  Port=3  Side=Left
  Motor 3 : PMIOPort  Port=4  Side=Left
  Motor 4 : PMIOPort  Port=5  Side=Left
  Body force : PMIOPort  Port=6  Side=Right
  Coil 1 Orientation : PMIOPort  Port=7  Side=Right
  Coil 2 Orientation : PMIOPort  Port=8  Side=Right
  Coil 3 Orientation : PMIOPort  Port=9  Side=Right
  Coil 4 Orientation : PMIOPort  Port=10  Side=Right
  wires:
  Constant/1 -> Simulink-PS Converter/1
  Constant1/1 -> Simulink-PS Converter1/1
  Constant2/1 -> Simulink-PS Converter2/1
  Constant3/1 -> Simulink-PS Converter3/1
  connections:
  ReferenceFrame/RConn1 -- F/RConn1 -- Rigid Transform6/LConn1 -- Rigid Transform4/LConn1 -- Rigid Transform2/LConn1 -- Rigid Transform/LConn1 -- Solid/RConn1
  Motor 1/RConn1 -- Coil 1 Orientation/RConn1 -- Solid/LConn1
  Coil 4 Orientation/RConn1 -- Motor 4/RConn1 -- Solid/LConn3
  Motor 2/RConn1 -- Coil 2 Orientation/RConn1 -- Solid/LConn2
  Coil 3 Orientation/RConn1 -- Motor 3/RConn1 -- Solid/RConn2
  Weld Joint/RConn1 -- Motor1/LConn1
  Rigid Transform/RConn1 -- Weld Joint/LConn1
  Rigid Transform1/LConn1 -- Motor1/RConn1
  Revolute Joint/LConn1 -- Rigid Transform1/RConn1
  Revolute Joint/RConn1 -- Propeller/LConn1
  Revolute Joint/LConn2 -- Simulink-PS Converter/RConn1
  Rigid Transform2/RConn1 -- Weld Joint1/LConn1
  Revolute Joint1/RConn1 -- Propeller1/LConn1
  Rigid Transform3/LConn1 -- Motor2/RConn1
  Revolute Joint1/LConn1 -- Rigid Transform3/RConn1
  Weld Joint1/RConn1 -- Motor2/LConn1
  Revolute Joint1/LConn2 -- Simulink-PS Converter1/RConn1
  Rigid Transform5/LConn1 -- Motors2/RConn1
  Weld Joint2/RConn1 -- Motors2/LConn1
  Revolute Joint2/LConn1 -- Rigid Transform5/RConn1
  Revolute Joint2/RConn1 -- Propeller2/LConn1
  Rigid Transform4/RConn1 -- Weld Joint2/LConn1
  Revolute Joint2/LConn2 -- Simulink-PS Converter2/RConn1
  Rigid Transform7/LConn1 -- Motors3/RConn1
  Weld Joint3/RConn1 -- Motors3/LConn1
  Revolute Joint3/LConn1 -- Rigid Transform7/RConn1
  Revolute Joint3/RConn1 -- Propeller3/LConn1
  Rigid Transform6/RConn1 -- Weld Joint3/LConn1
  Revolute Joint3/LConn2 -- Simulink-PS Converter3/RConn1
  Body force/RConn1 -- Solid/RConn3

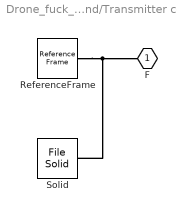
== system Drone_fuck_around/Transmitter coil ==
  ReferenceFrame : sm_lib/Frames and Transforms/Reference Frame
  Solid : sm_lib/Body Elements/File Solid  ExtGeomFileName=C:\Users\ivanb\OneDrive\Documents\Team 2261 Files\Mechanical Simulation\Transmitter coil Mk1_Default_sldprt.STEP  UnitType=FromFile  ExtGeomFileUnits=m  StepReaderType=HEX  ExportConvexHullGeometry=off  InertiaType=Custom  Mass=smiData.Solid(2).mass  MassUnits=kg  CenterOfMass=smiData.Solid(2).CoM  CenterOfMassUnits=in  MomentsOfInertia=smiData.Solid(2).MoI  MomentsOfInertiaUnits=kg*in^2  ProductsOfInertia=smiData.Solid(2).PoI  ProductsOfInertiaUnits=kg*in^2  BasedOnType=DensityFromFile  Density=1000  DensityUnits=kg/m^3  DoExposeReferenceFrame=on  SerializedFrames=<Frames/>  GraphicType=FromGeometry  MarkerShape=Sphere  MarkerSize=10  GraphicVisPropType=SimpleVisualProperties  GraphicDiffuseColor=smiData.Solid(2).color  GraphicSpecularColor=[0.5 0.5 0.5 1.0]  GraphicAmbientColor=[0.15 0.15 0.15 1.0]  GraphicEmissiveColor=[0.0 0.0 0.0 1.0]  GraphicShininess=75  GraphicOpacity=smiData.Solid(2).opacity
  F : PMIOPort  Side=Left
  connections:
  Solid/RConn1 -- ReferenceFrame/RConn1 -- F/RConn1

== matlab function Drone_fuck_around/MATLAB Function1 ==
  data: Rp input; M output; Rs input; pc input; n input; tol input
% function M=Babic_24(Rp,Rs,pc,n,tol)
%
% Returns the mutual inductance between two circular loops of radius Rp and Rs (with Rp >= Rs),
% whose centers are separated by a vector pc=[xc,yc,zc], and normal to the plane of secondary loop
% is n=[a,b,c], with absolute tolerance "tol" (default: 1e-10)
%
% All dimensions must be in "meters" and angles in "radians"
%
% The formula used in this function is the one provided by:
% S. Babic, F. Sirois, C. Akyel and C. Girardi, IEEE Trans. Magn., 2010, at press.
%
% The units have been adapted to the S.I. system
%
% Programmed by F. Sirois and S. Babic
% Ecole Polytechnique de Montreal, June 2009

function M=Babic_24(Rp,Rs,pc,n,tol)

if nargin==4,
   tol=1e-13;
elseif nargin<4 || nargin >5,
   error('Wrong number of parameters in function call (Babic_24.m)!');
end

% Recovery of parameters
xc=pc(1); yc=pc(2); zc=pc(3); 
a=n(1); b=n(2); c=n(3); 

% Preliminary computations
alpha=Rs/Rp; beta=xc/Rp; gamma=yc/Rp; delta=zc/Rp;

% Integration, Romberg method (adaptation from author below)
%   Author: Martin Kacenak,
%           Department of Informatics and Control Engineering,
%           Faculty of BERG, Technical University of Kosice,
%           B.Nemcovej 3, 04200 Kosice, Slovak Republic
%   E-mail: ma.kac@post.cz
%   Date:   february 2001
% (Any other numerical integration method would work as well)

decdigs=abs(floor(log10(tol)));
rom=zeros(2,decdigs);
romall=zeros(1,(2^(decdigs-1))+1);   



p = 0:2*pi/2^(decdigs-1):2*pi;
h = alpha;
e = beta;
g = gamma;
d = delta;


h2=h*h; e2=e*e; g2=g*g; a2=a*a; b2=b*b; c2=c*c;
l2=(a*a+c2); l=sqrt(l2); L2=(l2+b*b); L=sqrt(L2); l2L2=L2*l2; lL=l*L;
sp=sin(p); cp=cos(p); cp2=cp.*cp; sp2=sp.*sp;
if l==0,
  p1=0; p2=-g*sign(b); p3=0; p4=-e*sign(b); p5=d;
  V=sqrt( e2+g2+ h2*cp2-2*h*e*sign(b)*cp );
else
  p1=g*c/l; p2=-(e*l2+g*a*b)/lL; p3=h*c/L; p4=(g*l2-e*a*b-d*b*c)/lL; p5=(d*a-e*c)/l;
  V=sqrt( (e2+g2) + h2*( (1-b2*c2/l2L2)*cp2 + c2/l2*sp2 + a*b*c/(l2*L)*sin(2*p) ) - 2*h/lL*(e*a*b-g*l2)*cp - 2*h*e*c/l*sp );
end
A= (1+e2+g2+h2+d*d) + 2*h*(p4*cp+p5*sp);
m=4*V./(A+2*V); k=sqrt(m);
[K,E]=ellipke(m);
PSI=(1-0.5*m).*K-E;
romall=(p1*cp+p2*sp+p3).*PSI./(k.*V.^1.5);




h=2*pi;
rom(1,1)=h*(romall(1)+romall(end))/2;
for i=2:decdigs
   step=2^(decdigs-i+1);
   % trapezoidal approximations
   rom(2,1)=(rom(1,1)+h*sum(romall((step/2)+1:step:2^(decdigs-1))))/2;
   % Richardson extrapolation
   for k=1:i-1
      rom(2,k+1)=((4^k)*rom(2,k)-rom(1,k))/((4^k)-1);
   end
   rom(1,1:i)=rom(2,1:i);
   h=h/2;
end
M=4e-7*Rs*rom(1,decdigs);

%%%%%%%%%%%%%%%%%%%%%%%%%%%%%%%%%%%%%%%%%%%%%%%%%%%%%%%%%%%%%%%%%%%%%%%%%%%%%%%%
% Integrand function

== matlab function Drone_fuck_around/Angle & Axs to RotMatrix1 ==
  data: alpha input; u input; R output; v input
function R = RotMatrix(alpha, u, v)
% RotMatrix - N-dimensional Rotation matrix
% R = RotMatrix(alpha, u, v)
% INPUT:
%   alpha: Angle of rotation in radians, counter-clockwise direction.
%   u, v:  If just the input alpha is provided, a 2D matrix is replied.
%          For 1 input u, the 3D rotation matrix is created. u must have 3
%          elements.
%          If u and v are used as inputs, the N-dimensional rotation is
%          performed in the hyperplane spanned by u and v. Note, that there is
%          no unique axis of rotation in N>3 dimensions.
%          u and v are normalized automatically and in the N-D case v is made
%          orthogonal to u.
%          The dimension of u and v determine the dimension of the output.
% OUTPUT:
%   R:     Rotation matrix.
%
% REFERENCES:
% analyticphysics.com/Higher%20Dimensions/Rotations%20in%20Higher%20Dimensions.htm
% en.wikipedia.org/wiki/Rotation_matrix
% application.wiley-vch.de/books/sample/3527406204_c01.pdf
%
% Tested: Matlab 2009a, 2015b(32/64), 2016b, 2018b, Win7/10
% Author: Jan Simon, Heidelberg, (C) 2018-2022 j@n-simon.de

% $JRev: R-e V:004 Sum:WqAShRoLB3Tk Date:30-Sep-2022 10:17:48 $
% $License: BSD (use/copy/change/redistribute on own risk, mention the author) $
% $File: Tools\GL3D\RotMatrix.m $
% History:
% 001: 10-Mar-2018 14:31, First version.
% 003: 30-Sep-2022 09:54, Typos fixed in comments.

% Initialize: ==================================================================
% Global Interface: ------------------------------------------------------------
% Initial values: --------------------------------------------------------------
% Program Interface: -----------------------------------------------------------
if numel(alpha) ~= 1
   error('JSimon:RotMatrrix:BadInput1', ...
      'Angle of rotation must be a scalar.');
end

% User Interface: --------------------------------------------------------------
% Do the work: =================================================================
s = sin(alpha);
c = cos(alpha);


if numel(u) ~= 3
         error('JSimon:RotMatrix:BadAxis2D', ...
            '3D: Rotation axis must have 3 elements.');
end

% Normalized vector:
u = u(:);
u = u ./ sqrt(u.' * u);
    
% 3D rotation matrix:
x  = u(1);
y  = u(2);
z  = u(3);
mc = 1 - c;
R  = [c + x * x * mc,      x * y * mc - z * s,   x * z * mc + y * s; ...
    x * y * mc + z * s,  c + y * y * mc,       y * z * mc - x * s; ...
    x * z * mc - y * s,  y * z * mc + x * s,   c + z * z .* mc];
         

end

== matlab function Drone_fuck_around/MATLAB Function2 ==
  data: Rp input; M output; Rs input; pc input; n input; tol input
% function M=Babic_24(Rp,Rs,pc,n,tol)
%
% Returns the mutual inductance between two circular loops of radius Rp and Rs (with Rp >= Rs),
% whose centers are separated by a vector pc=[xc,yc,zc], and normal to the plane of secondary loop
% is n=[a,b,c], with absolute tolerance "tol" (default: 1e-10)
%
% All dimensions must be in "meters" and angles in "radians"
%
% The formula used in this function is the one provided by:
% S. Babic, F. Sirois, C. Akyel and C. Girardi, IEEE Trans. Magn., 2010, at press.
%
% The units have been adapted to the S.I. system
%
% Programmed by F. Sirois and S. Babic
% Ecole Polytechnique de Montreal, June 2009

function M=Babic_24(Rp,Rs,pc,n,tol)

if nargin==4,
   tol=1e-13;
elseif nargin<4 || nargin >5,
   error('Wrong number of parameters in function call (Babic_24.m)!');
end

% Recovery of parameters
xc=pc(1); yc=pc(2); zc=pc(3); 
a=n(1); b=n(2); c=n(3); 

% Preliminary computations
alpha=Rs/Rp; beta=xc/Rp; gamma=yc/Rp; delta=zc/Rp;

% Integration, Romberg method (adaptation from author below)
%   Author: Martin Kacenak,
%           Department of Informatics and Control Engineering,
%           Faculty of BERG, Technical University of Kosice,
%           B.Nemcovej 3, 04200 Kosice, Slovak Republic
%   E-mail: ma.kac@post.cz
%   Date:   february 2001
% (Any other numerical integration method would work as well)

decdigs=abs(floor(log10(tol)));
rom=zeros(2,decdigs);
romall=zeros(1,(2^(decdigs-1))+1);   






p = 0:2*pi/2^(decdigs-1):2*pi;
h = alpha;
e = beta;
g = gamma;
d = delta;


h2=h*h; e2=e*e; g2=g*g; a2=a*a; b2=b*b; c2=c*c;
l2=(a*a+c2); l=sqrt(l2); L2=(l2+b*b); L=sqrt(L2); l2L2=L2*l2; lL=l*L;
sp=sin(p); cp=cos(p); cp2=cp.*cp; sp2=sp.*sp;
if l==0,
  p1=0; p2=-g*sign(b); p3=0; p4=-e*sign(b); p5=d;
  V=sqrt( e2+g2+ h2*cp2-2*h*e*sign(b)*cp );
else
  p1=g*c/l; p2=-(e*l2+g*a*b)/lL; p3=h*c/L; p4=(g*l2-e*a*b-d*b*c)/lL; p5=(d*a-e*c)/l;
  V=sqrt( (e2+g2) + h2*( (1-b2*c2/l2L2)*cp2 + c2/l2*sp2 + a*b*c/(l2*L)*sin(2*p) ) - 2*h/lL*(e*a*b-g*l2)*cp - 2*h*e*c/l*sp );
end
A= (1+e2+g2+h2+d*d) + 2*h*(p4*cp+p5*sp);
m=4*V./(A+2*V); k=sqrt(m);
[K,E]=ellipke(m);
PSI=(1-0.5*m).*K-E;
romall=(p1*cp+p2*sp+p3).*PSI./(k.*V.^1.5);



h=2*pi;
rom(1,1)=h*(romall(1)+romall(end))/2;
for i=2:decdigs
   step=2^(decdigs-i+1);
   % trapezoidal approximations
   rom(2,1)=(rom(1,1)+h*sum(romall((step/2)+1:step:2^(decdigs-1))))/2;
   % Richardson extrapolation
   for k=1:i-1
      rom(2,k+1)=((4^k)*rom(2,k)-rom(1,k))/((4^k)-1);
   end
   rom(1,1:i)=rom(2,1:i);
   h=h/2;
end
M=4e-7*Rs*rom(1,decdigs);

%%%%%%%%%%%%%%%%%%%%%%%%%%%%%%%%%%%%%%%%%%%%%%%%%%%%%%%%%%%%%%%%%%%%%%%%%%%%%%%%
% Integrand function
